simulink model "ABS__"  (R2018b)
settings: Solver=VariableStepAuto  StartTime=0.0  StopTime=5  RelTol=1e-3
values from neighbouring files (symbols this model uses):
  Cfr = 0.35    [Autotronics.m]
  Dmc = 0.018    [Autotronics.m]
  Dwc = 0.055    [Autotronics.m]
  Fh = 100    [Autotronics.m]
  K = 3.75    [Autotronics.m]
  m = 1700    [Autotronics.m]
  V0 = V0 / 3.6    (= 27.7777777778)    [Autotronics.m]
  W = m * 9.81    (= 16677)    [Autotronics.m]
undefined symbols (not defined in the file or in its folder): inertia, sigbuilder_block
settings Model: Creator=Aly  LastModifiedBy=Aly

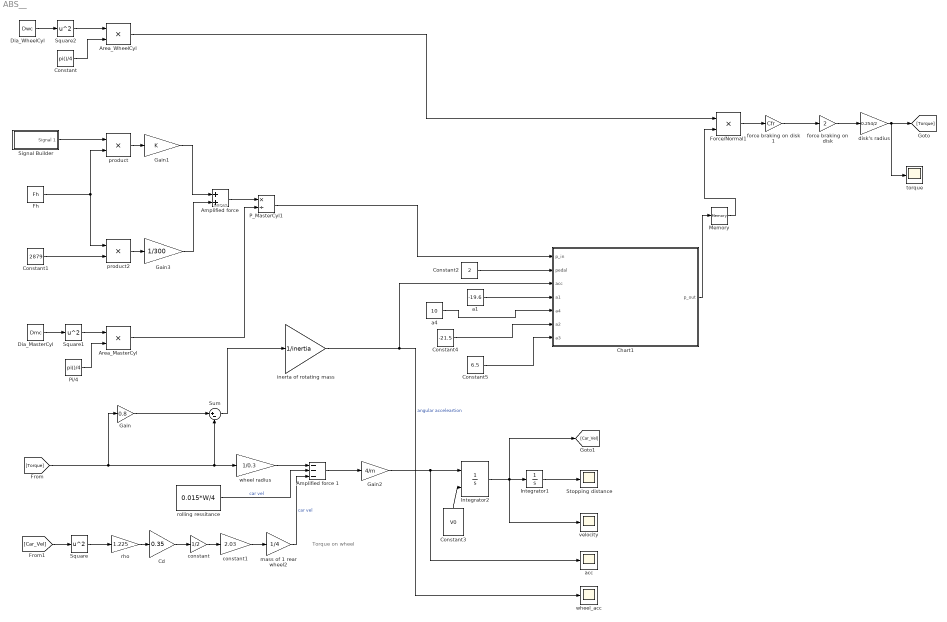
== system ABS__ ==
  note: servo
  note: Torque on wheel
  "Amplified force " : Sum
  Amplified force 1 : Sum  Inputs=---
  Area_MasterCyl : Product
  Area_WheelCyl : Product
  Cd : Gain  Gain=0.35
  Chart1 : Stateflow chart  TreatAsAtomicUnit=on
  Constant : Constant  Value=pi()/4
  Constant1 : Constant  Value=2879
  Constant2 : Constant  Value=2
  Constant3 : Constant  Value=V0
  Constant4 : Constant  Value=-21.5
  Constant5 : Constant  Value=6.5
  Dia_MasterCyl : Constant  Value=Dmc
  Dia_WheelCyl : Constant  Value=Dwc
  Fh : Constant  Value=Fh
  Force/Normal1 : Product
  Gain : Gain  Gain=0.8
  Gain1 : Gain  Gain=K
  Gain2 : Gain  Gain=4/m
  Gain3 : Gain  Gain=1/300
  Integrator1 : Integrator
  Integrator2 : Integrator  InitialConditionSource=external  InitialCondition=27.7  LimitOutput=on  UpperSaturationLimit=27.7  LowerSaturationLimit=0
  Memory : Memory
  P_MasterCyl1 : Product  Inputs=*/
  Pi/4 : Constant  Value=pi()/4
  Signal Builder : Subsystem  Tag=STV Subsys  LoadFcn=sigbuilder_block('load');  StartFcn=sigbuilder_block('start');  StopFcn=sigbuilder_block('stop');  ClipboardFcn=sigbuilder_block('clipboard');  mask(Sigbuilder block){tuvar=[0:10]}
      mask help: Simulink:masks:SigbuilderBlock_MD
      mask init:
      | if ~strcmp(get_param(bdroot(gcbh),'SimulationStatus'),'stopped') tuvar = sigbuilder_block('maskInit'); end
      settings: CopyFcn=sigbuilder_block('copy');  DeleteFcn=sigbuilder_block('delete');  ModelCloseFcn=sigbuilder_block('modelClose');  PreSaveFcn=sigbuilder_block('preSave');  PauseFcn=sigbuilder_block('pause');  ContinueFcn=sigbuilder_block('continue');  NameChangeFcn=sigbuilder_block('namechange');  OpenFcn=sigbuilder_block('open',[0 0 978 518.25 ]);  CloseFcn=sigbuilder_block('close');
      mask Display: plot(0, 0, 100, 100,[2, 2, 32, 32, 2], [68, 8, 8, 68, 68],[32, 2], [38, 38], [32, 19, 2],[53, 60, 44], [32, 17, 17, 2],[16, 16, 31, 31]);txt = getActiveGroup(gcbh);text(2, 100, txt,'verticalAlignment', 'top');
  Square : Math  Operator=square  SaturateOnIntegerOverflow=on
  Square1 : Math  Operator=square  OutputSignalType=real  SaturateOnIntegerOverflow=on
  Square2 : Math  Operator=square  OutputSignalType=real  SaturateOnIntegerOverflow=on
  Stopping distance : Scope
  Sum : Sum  Inputs=|+-
  a1 : Constant  Value=-19.6
  a4 : Constant  Value=10
  acc : Scope
  constant : Gain  Gain=1/2
  constant1 : Gain  Gain=2.03
  disk's radius : Gain  Gain=0.254/2
  "force braking on disk " : Gain  Gain=2
  force braking on disk 1 : Gain  Gain=Cfr
  inerta of rotating mass : Gain  Gain=1/inertia
  mass of 1 rear wheel2 : Gain  Gain=1/4
  product : Product
  product2 : Product
  rho : Gain  Gain=1.225
  rolling ressitance : Constant  Value=0.015*W/4
  torque : Scope
  "velocity " : Scope
  wheel radius : Gain  Gain=1/0.3
  wheel_acc : Scope
  wires:
  [Car_Vel] -> Square/1
  rho/1 -> Cd/1
  Memory/1 -> Force/Normal1/2
  a4/1 -> Chart1/5(a4)
  Constant4/1 -> Chart1/6(a2)
  P_MasterCyl1/1 -> Chart1/1(p_in)
  Area_WheelCyl/1 -> Force/Normal1/1
  [Torque] -> Gain/1, Sum/2, wheel radius/1
  mass of 1 rear wheel2/1 -> Amplified force 1/3  "car vel"
  Chart1/1(p_out) -> Memory/1
  inerta of rotating mass/1 -> Chart1/3(acc), wheel_acc/1  "angular acceleartion"
  Constant3/1 -> Integrator2/2
  Pi/4/1 -> Area_MasterCyl/2
  Signal Builder/1(Signal 1) -> product/1
  rolling ressitance/1 -> Amplified force 1/2  "car vel"
  Constant1/1 -> product2/2
  Constant2/1 -> Chart1/2(pedal)
  product/1 -> Gain1/1
  Fh/1 -> product/2, product2/1
  Integrator2/1 -> [Car_Vel], "velocity "/1, Integrator1/1
  "Amplified force "/1 -> P_MasterCyl1/1
  Area_MasterCyl/1 -> P_MasterCyl1/2
  constant1/1 -> mass of 1 rear wheel2/1
  disk's radius/1 -> torque/1, [Torque]
  a1/1 -> Chart1/4(a1)
  force braking on disk 1/1 -> "force braking on disk "/1
  Gain3/1 -> "Amplified force "/2
  Square/1 -> rho/1
  wheel radius/1 -> Amplified force 1/1
  Amplified force 1/1 -> Gain2/1
  Dia_MasterCyl/1 -> Square1/1
  Constant/1 -> Area_WheelCyl/2
  Dia_WheelCyl/1 -> Square2/1
  constant/1 -> constant1/1
  Square1/1 -> Area_MasterCyl/1
  Constant5/1 -> Chart1/7(a3)
  Force/Normal1/1 -> force braking on disk 1/1
  product2/1 -> Gain3/1
  Integrator1/1 -> Stopping distance/1
  Sum/1 -> inerta of rotating mass/1
  "force braking on disk "/1 -> disk's radius/1
  Gain2/1 -> acc/1, Integrator2/1
  Square2/1 -> Area_WheelCyl/1
  Gain1/1 -> "Amplified force "/1
  Cd/1 -> constant/1
  Gain/1 -> Sum/1

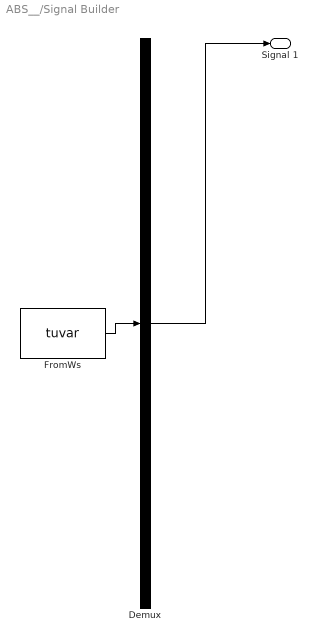
== system ABS__/Signal Builder ==
  Demux : Demux  Tag=STV Demux  Outputs=1
  FromWs : FromWorkspace  Tag=STV FromWs  VariableName=tuvar  SampleTime=0
      SigBuilderData=|
      | common.afterFinalStr = 'Extrapolate'
      | common.sampleTime = 0
      | dataSet.timeRange = [0 10]
      | dataSet.name = 'Group 1'
      | sbobj.Groups.Name = 'Group 1'
      | sbobj.Groups.Signals.Name = 'Signal 1'
      | sbobj.Groups.Signals.XData = [0 0.5 10]
      | sbobj.Groups.Signals.YData = [0.005 1 0.995]
  Signal 1 : Outport  Tag=STV Outport
  wires:
  Demux/1 -> Signal 1/1
  FromWs/1 -> Demux/1

== stateflow chart ABS__/Chart1 ==
  state Released
  state state1
    during:
    p_out=p_out*1.1
  state passive
    entry:p_out=p_in
  state state2
    during:
    p_out=p_out*1.01
  state state3
    during:
    p_out=p_out/1.1
  state state4
    during:
    p_out=p_out/2
  state state5
    entry:
    p_out=p_out*1.1
  (default) -> Released
  state1 -> passive [order 2] : [pedal<0.2]
  Released -> passive : [pedal > 0.02]
  state1 -> state2 [order 1] : [acc<a1]
  passive -> Released [order 2] : [pedal<0.02]
  passive -> state1 [order 1] : [pedal>0.8]
  state2 -> state3 : [ acc<a2]
  state3 -> state4 : [acc>a1]
  state4 -> state5 : [acc>a4]
  data: p_in input; pedal input; acc input; p_out output; a1 input; a4 input; a2 input; a3 input
